simulink model "ackerman_ROS_neural_controller_v2"  (R2023a)
settings: Solver=FixedStepDiscrete  StartTime=0.0  StopTime=200  FixedStep=0.1  RelTol=1e-3
undefined symbols (not defined in the file or in its folder): Angular, Linear
libraries: neural x413, robotlib x15, robotcorelib x1
(part 11 of 17)

== system ackerman_ROS_neural_controller_v2/casi 3 - 15 20 15/Layer 1/IW{1,1} ==
  "pd{1,1}" : Inport  PortDimensions=8  SampleTime=0.1
      mask Display: e = 0.06;c1 = [120 230 180]/255;c2 = ([120 230 180]+0)/(256+128);c3 = ([120 230 180]+128)/(256+128);patch([0 1 1 0],[0 0 1 1],c1);patch([0 1 1 1-e 1-e 0+e],[0 0 1 1-e 0+e 0+e],c2);patch([0 0 1 1-e 0+e 0+e],[0 1 1 1-e 1-e 0+e],c3);plot([0 1 1 0 0],[0 0 1 1 0]);
  "IW{1,1}(1,:)'" : Constant  Value=[2.897737054776072351813809291343204677104949951171875;-0.97777917153495874647006758095812983810901641845703125;-1.95913475138207981984805883257649838924407958984375;3.442897344122934466525975949480198323726654052734375;-7.99002240223826820653130198479630053043365478515625;1.271756533327842220160164288245141506195068359375;5.08245618160992140843745801248587667942047119140625;-9.02719443592735615311539731919765472412109375]
      mask Display: e = 0.06;c1 = [120 150 230]/255;c2 = ([120 150 230]+0)/383;c3 = ([120 150 230]+128)/383;patch([0 1 1 0],[0 0 1 1],c1);patch([0 1 1 1-e 1-e 0+e],[0 0 1 1-e 0+e 0+e],c2);patch([0 0 1 1-e 0+e 0+e],[0 1 1 1-e 1-e 0+e],c3);plot([0 1 1 0 0],[0 0 1 1 0]);disp('Weights');
  "IW{1,1}(10,:)'" : Constant  Value=[-0.82593178229890984454186764196492731571197509765625;2.35210993951447111527386368834413588047027587890625;0.292170459956925199218602529072086326777935028076171875;-1.0114862071536403487215238783392123878002166748046875;-4.12104019955256095641971114673651754856109619140625;-0.81766281683690511528084243764169514179229736328125;1.8519098472877104644140899836202152073383331298828125;-1.116663125058864114436119052697904407978057861328125]
      mask Display: e = 0.06;c1 = [120 150 230]/255;c2 = ([120 150 230]+0)/383;c3 = ([120 150 230]+128)/383;patch([0 1 1 0],[0 0 1 1],c1);patch([0 1 1 1-e 1-e 0+e],[0 0 1 1-e 0+e 0+e],c2);patch([0 0 1 1-e 0+e 0+e],[0 1 1 1-e 1-e 0+e],c3);plot([0 1 1 0 0],[0 0 1 1 0]);disp('Weights');
  "IW{1,1}(11,:)'" : Constant  Value=[-0.078503432809702233807769289342104457318782806396484375;-1.31700463726781347162386737181805074214935302734375;-1.91049666805551243697891550255008041858673095703125;1.4172024682093269376537136849947273731231689453125;-3.09796436612653902642477987683378159999847412109375;-0.98792077372010644875643947671051137149333953857421875;-0.01101359556692830914126357555460344883613288402557373046875;-1.895967746941914722214050925686024129390716552734375]
      mask Display: e = 0.06;c1 = [120 150 230]/255;c2 = ([120 150 230]+0)/383;c3 = ([120 150 230]+128)/383;patch([0 1 1 0],[0 0 1 1],c1);patch([0 1 1 1-e 1-e 0+e],[0 0 1 1-e 0+e 0+e],c2);patch([0 0 1 1-e 0+e 0+e],[0 1 1 1-e 1-e 0+e],c3);plot([0 1 1 0 0],[0 0 1 1 0]);disp('Weights');
  "IW{1,1}(12,:)'" : Constant  Value=[-0.8106197384996172150550819424097426235675811767578125;-0.6227986203077999771693384900572709739208221435546875;1.0411180629325134106011319090612232685089111328125;0.6012357382346260603611654005362652242183685302734375;-1.1876488848888768767864121400634758174419403076171875;-2.475733573131647435872082496643997728824615478515625;-1.7927537050774613458514750163885764777660369873046875;-0.999271370716360962660473887808620929718017578125]
      mask Display: e = 0.06;c1 = [120 150 230]/255;c2 = ([120 150 230]+0)/383;c3 = ([120 150 230]+128)/383;patch([0 1 1 0],[0 0 1 1],c1);patch([0 1 1 1-e 1-e 0+e],[0 0 1 1-e 0+e 0+e],c2);patch([0 0 1 1-e 0+e 0+e],[0 1 1 1-e 1-e 0+e],c3);plot([0 1 1 0 0],[0 0 1 1 0]);disp('Weights');
  "IW{1,1}(13,:)'" : Constant  Value=[1.9200847723387510779247122627566568553447723388671875;1.7864125475128134201696639138390310108661651611328125;-2.619916383345554766748364272643812000751495361328125;-0.368745431713104476756370786461047828197479248046875;-1.7276054344216331681849396773031912744045257568359375;1.2160295695674230298521933946176432073116302490234375;0.266643899945036511045515226214774884283542633056640625;-2.80681458166946651289208602975122630596160888671875]
      mask Display: e = 0.06;c1 = [120 150 230]/255;c2 = ([120 150 230]+0)/383;c3 = ([120 150 230]+128)/383;patch([0 1 1 0],[0 0 1 1],c1);patch([0 1 1 1-e 1-e 0+e],[0 0 1 1-e 0+e 0+e],c2);patch([0 0 1 1-e 0+e 0+e],[0 1 1 1-e 1-e 0+e],c3);plot([0 1 1 0 0],[0 0 1 1 0]);disp('Weights');
  "IW{1,1}(14,:)'" : Constant  Value=[0.9980731449312667535878063063137233257293701171875;-3.114409533087536541273721013567410409450531005859375;0.45617718431620690733296896723913960158824920654296875;-4.31118482402145541954041618737392127513885498046875;0.75844871154216975117634547132183797657489776611328125;4.07356626581029690470359128084965050220489501953125;-0.18504498285524795253564889208064414560794830322265625;0.840293231307919885608725962811149656772613525390625]
      mask Display: e = 0.06;c1 = [120 150 230]/255;c2 = ([120 150 230]+0)/383;c3 = ([120 150 230]+128)/383;patch([0 1 1 0],[0 0 1 1],c1);patch([0 1 1 1-e 1-e 0+e],[0 0 1 1-e 0+e 0+e],c2);patch([0 0 1 1-e 0+e 0+e],[0 1 1 1-e 1-e 0+e],c3);plot([0 1 1 0 0],[0 0 1 1 0]);disp('Weights');
  "IW{1,1}(15,:)'" : Constant  Value=[0.264348557935919270533986491500400006771087646484375;1.6376069116661342572882631429820321500301361083984375;0.54287049402263531927559370160452090203762054443359375;-1.536888279368743059905000336584635078907012939453125;-1.511976681548248269137957322527654469013214111328125;-1.110912669638801641980307977064512670040130615234375;0.323317174054256251114480846808874048292636871337890625;0.49728314679400742459591810984420590102672576904296875]
      mask Display: e = 0.06;c1 = [120 150 230]/255;c2 = ([120 150 230]+0)/383;c3 = ([120 150 230]+128)/383;patch([0 1 1 0],[0 0 1 1],c1);patch([0 1 1 1-e 1-e 0+e],[0 0 1 1-e 0+e 0+e],c2);patch([0 0 1 1-e 0+e 0+e],[0 1 1 1-e 1-e 0+e],c3);plot([0 1 1 0 0],[0 0 1 1 0]);disp('Weights');
  "IW{1,1}(2,:)'" : Constant  Value=[-4.26598336004146716504692449234426021575927734375;-0.0716533501066898559361817433455144055187702178955078125;1.3698494058938184281259964336641132831573486328125;1.0032592579538570642938566379598341882228851318359375;0.1350385776637200996308507683352218009531497955322265625;3.6066214754247578611057178932242095470428466796875;-2.493648707013484955297144551877863705158233642578125;-1.2915573005255687188963520384277217090129852294921875]
      mask Display: e = 0.06;c1 = [120 150 230]/255;c2 = ([120 150 230]+0)/383;c3 = ([120 150 230]+128)/383;patch([0 1 1 0],[0 0 1 1],c1);patch([0 1 1 1-e 1-e 0+e],[0 0 1 1-e 0+e 0+e],c2);patch([0 0 1 1-e 0+e 0+e],[0 1 1 1-e 1-e 0+e],c3);plot([0 1 1 0 0],[0 0 1 1 0]);disp('Weights');
  "IW{1,1}(3,:)'" : Constant  Value=[-2.444535165218435945888586502405814826488494873046875;-1.50490350149213014674387522973120212554931640625;0.06968386498528870987012595605847309343516826629638671875;-0.763333843294209390961668759700842201709747314453125;-3.419767268873754151314869886846281588077545166015625;3.115085244912598749777998818899504840373992919921875;0.60136703915281997101516253678710199892520904541015625;1.74995131625876876313441243837587535381317138671875]
      mask Display: e = 0.06;c1 = [120 150 230]/255;c2 = ([120 150 230]+0)/383;c3 = ([120 150 230]+128)/383;patch([0 1 1 0],[0 0 1 1],c1);patch([0 1 1 1-e 1-e 0+e],[0 0 1 1-e 0+e 0+e],c2);patch([0 0 1 1-e 0+e 0+e],[0 1 1 1-e 1-e 0+e],c3);plot([0 1 1 0 0],[0 0 1 1 0]);disp('Weights');
  "IW{1,1}(4,:)'" : Constant  Value=[-0.64761712625556200340071200116653926670551300048828125;-0.31853889917769662165625277339131571352481842041015625;1.51716786863737151946907033561728894710540771484375;-4.5277687962268426957734845927916467189788818359375;-2.555852630048429663389697452657856047153472900390625;2.557007613553910818637859847513027489185333251953125;0.8989737939253752418977683191769756376743316650390625;0.85350327193705055606187670491635799407958984375]
      mask Display: e = 0.06;c1 = [120 150 230]/255;c2 = ([120 150 230]+0)/383;c3 = ([120 150 230]+128)/383;patch([0 1 1 0],[0 0 1 1],c1);patch([0 1 1 1-e 1-e 0+e],[0 0 1 1-e 0+e 0+e],c2);patch([0 0 1 1-e 0+e 0+e],[0 1 1 1-e 1-e 0+e],c3);plot([0 1 1 0 0],[0 0 1 1 0]);disp('Weights');
  "IW{1,1}(5,:)'" : Constant  Value=[0.0600879788316249496826770837287767790257930755615234375;2.548876161006494722727211410528980195522308349609375;-0.89919509804499553329293348724604584276676177978515625;0.39216783743824390473520224986714310944080352783203125;1.803154797478246695874304350581951439380645751953125;0.670064472196073790399850622634403407573699951171875;0.279308252151045988131983222046983428299427032470703125;-1.9897152695475430750349232766893692314624786376953125]
      mask Display: e = 0.06;c1 = [120 150 230]/255;c2 = ([120 150 230]+0)/383;c3 = ([120 150 230]+128)/383;patch([0 1 1 0],[0 0 1 1],c1);patch([0 1 1 1-e 1-e 0+e],[0 0 1 1-e 0+e 0+e],c2);patch([0 0 1 1-e 0+e 0+e],[0 1 1 1-e 1-e 0+e],c3);plot([0 1 1 0 0],[0 0 1 1 0]);disp('Weights');
  "IW{1,1}(6,:)'" : Constant  Value=[1.516320780958766878399046618142165243625640869140625;-1.15730560900975998350759255117736756801605224609375;0.458524114660376624907911491391132585704326629638671875;-1.102990345663160010047931791632436215877532958984375;2.2751191767257754605680020176805555820465087890625;0.26970804091846589667369471499114297330379486083984375;0.009118671069833252096348275017589912749826908111572265625;0.030751765387002298612895145879519986920058727264404296875]
      mask Display: e = 0.06;c1 = [120 150 230]/255;c2 = ([120 150 230]+0)/383;c3 = ([120 150 230]+128)/383;patch([0 1 1 0],[0 0 1 1],c1);patch([0 1 1 1-e 1-e 0+e],[0 0 1 1-e 0+e 0+e],c2);patch([0 0 1 1-e 0+e 0+e],[0 1 1 1-e 1-e 0+e],c3);plot([0 1 1 0 0],[0 0 1 1 0]);disp('Weights');
  "IW{1,1}(7,:)'" : Constant  Value=[1.0256630959773380684652011041180230677127838134765625;0.953736010400195066694095658021979033946990966796875;0.91140415232379068388723908356041647493839263916015625;0.07112913381762824005516421266293036751449108123779296875;1.7300742608625514495912511847564019262790679931640625;-1.3492253267064329147473245029686950147151947021484375;1.091559740272355583101671072654426097869873046875;0.1343110570666319336652350102667696774005889892578125]
      mask Display: e = 0.06;c1 = [120 150 230]/255;c2 = ([120 150 230]+0)/383;c3 = ([120 150 230]+128)/383;patch([0 1 1 0],[0 0 1 1],c1);patch([0 1 1 1-e 1-e 0+e],[0 0 1 1-e 0+e 0+e],c2);patch([0 0 1 1-e 0+e 0+e],[0 1 1 1-e 1-e 0+e],c3);plot([0 1 1 0 0],[0 0 1 1 0]);disp('Weights');
  "IW{1,1}(8,:)'" : Constant  Value=[-0.46823002994979656676832746597938239574432373046875;-2.389488306025070674110111212939955294132232666015625;1.19212611072083252139464093488641083240509033203125;0.203108224876829390748156356494291685521602630615234375;-3.12759889820417225081428114208392798900604248046875;-4.1826406226244738917330323602072894573211669921875;-0.83564532349110642872602738862042315304279327392578125;0.24560268558538178584882416544132865965366363525390625]
      mask Display: e = 0.06;c1 = [120 150 230]/255;c2 = ([120 150 230]+0)/383;c3 = ([120 150 230]+128)/383;patch([0 1 1 0],[0 0 1 1],c1);patch([0 1 1 1-e 1-e 0+e],[0 0 1 1-e 0+e 0+e],c2);patch([0 0 1 1-e 0+e 0+e],[0 1 1 1-e 1-e 0+e],c3);plot([0 1 1 0 0],[0 0 1 1 0]);disp('Weights');
  "IW{1,1}(9,:)'" : Constant  Value=[0.1263911266086849838341521490292507223784923553466796875;0.0566874449298560012522329998319037258625030517578125;1.8401514119086339604791646706871688365936279296875;0.528937864859507111958691893960349261760711669921875;3.9851213758785686280816662474535405635833740234375;-1.5845796502176010545070994339766912162303924560546875;0.82335138653403949771103498278534971177577972412109375;-0.1356210234756699828384540751358144916594028472900390625]
      mask Display: e = 0.06;c1 = [120 150 230]/255;c2 = ([120 150 230]+0)/383;c3 = ([120 150 230]+128)/383;patch([0 1 1 0],[0 0 1 1],c1);patch([0 1 1 1-e 1-e 0+e],[0 0 1 1-e 0+e 0+e],c2);patch([0 0 1 1-e 0+e 0+e],[0 1 1 1-e 1-e 0+e],c3);plot([0 1 1 0 0],[0 0 1 1 0]);disp('Weights');
  Mux : Mux  Inputs=15
      mask Display: e = 0.06;c1 = [120 150 230]/255;c2 = ([120 150 230]+0)/383;c3 = ([120 150 230]+128)/383;patch([0 1 1 0],[0 0 1 1],c1);patch([0 1 1 1-e 1-e 0+e],[0 0 1 1-e 0+e 0+e],c2);patch([0 0 1 1-e 0+e 0+e],[0 1 1 1-e 1-e 0+e],c3);plot([0 1 1 0 0],[0 0 1 1 0]);disp('Mux');
  dotprod{1..15} (15 alike) : neural/Weight Functions/dotprod
  "iz{1,1}" : Outport
      mask Display: e = 0.06;c1 = [120 230 180]/255;c2 = ([120 230 180]+0)/(256+128);c3 = ([120 230 180]+128)/(256+128);patch([0 1 1 0],[0 0 1 1],c1);patch([0 1 1 1-e 1-e 0+e],[0 0 1 1-e 0+e 0+e],c2);patch([0 0 1 1-e 0+e 0+e],[0 1 1 1-e 1-e 0+e],c3);plot([0 1 1 0 0],[0 0 1 1 0]);
  wires:
  "IW{1,1}(1,:)'"/1 -> dotprod1/1
  "pd{1,1}"/1 -> dotprod1/2, dotprod2/2, dotprod3/2, dotprod4/2, dotprod5/2, dotprod6/2, dotprod7/2, dotprod8/2, dotprod9/2, dotprod10/2, dotprod11/2, dotprod12/2, dotprod13/2, dotprod14/2, dotprod15/2
  dotprod1/1 -> Mux/1
  "IW{1,1}(2,:)'"/1 -> dotprod2/1
  dotprod2/1 -> Mux/2
  "IW{1,1}(3,:)'"/1 -> dotprod3/1
  dotprod3/1 -> Mux/3
  "IW{1,1}(4,:)'"/1 -> dotprod4/1
  dotprod4/1 -> Mux/4
  "IW{1,1}(5,:)'"/1 -> dotprod5/1
  dotprod5/1 -> Mux/5
  "IW{1,1}(6,:)'"/1 -> dotprod6/1
  dotprod6/1 -> Mux/6
  "IW{1,1}(7,:)'"/1 -> dotprod7/1
  dotprod7/1 -> Mux/7
  "IW{1,1}(8,:)'"/1 -> dotprod8/1
  dotprod8/1 -> Mux/8
  "IW{1,1}(9,:)'"/1 -> dotprod9/1
  dotprod9/1 -> Mux/9
  "IW{1,1}(10,:)'"/1 -> dotprod10/1
  dotprod10/1 -> Mux/10
  "IW{1,1}(11,:)'"/1 -> dotprod11/1
  dotprod11/1 -> Mux/11
  "IW{1,1}(12,:)'"/1 -> dotprod12/1
  dotprod12/1 -> Mux/12
  "IW{1,1}(13,:)'"/1 -> dotprod13/1
  dotprod13/1 -> Mux/13
  "IW{1,1}(14,:)'"/1 -> dotprod14/1
  dotprod14/1 -> Mux/14
  "IW{1,1}(15,:)'"/1 -> dotprod15/1
  dotprod15/1 -> Mux/15
  Mux/1 -> "iz{1,1}"/1

== system ackerman_ROS_neural_controller_v2/casi 3 - 15 20 15/Layer 2/Delays 1 ==
  "p{2}" : Inport  PortDimensions=15  SampleTime=0.1
      mask Display: e = 0.06;c1 = [120 230 180]/255;c2 = ([120 230 180]+0)/(256+128);c3 = ([120 230 180]+128)/(256+128);patch([0 1 1 0],[0 0 1 1],c1);patch([0 1 1 1-e 1-e 0+e],[0 0 1 1-e 0+e 0+e],c2);patch([0 0 1 1-e 0+e 0+e],[0 1 1 1-e 1-e 0+e],c3);plot([0 1 1 0 0],[0 0 1 1 0]);
  mux : Mux  Inputs=1
      mask Display: e = 0.06;c1 = [120 150 230]/255;c2 = ([120 150 230]+0)/383;c3 = ([120 150 230]+128)/383;patch([0 1 1 0],[0 0 1 1],c1);patch([0 1 1 1-e 1-e 0+e],[0 0 1 1-e 0+e 0+e],c2);patch([0 0 1 1-e 0+e 0+e],[0 1 1 1-e 1-e 0+e],c3);plot([0 1 1 0 0],[0 0 1 1 0]);disp('Mux')
  "pd{2,1}" : Outport
      mask Display: e = 0.06;c1 = [120 230 180]/255;c2 = ([120 230 180]+0)/(256+128);c3 = ([120 230 180]+128)/(256+128);patch([0 1 1 0],[0 0 1 1],c1);patch([0 1 1 1-e 1-e 0+e],[0 0 1 1-e 0+e 0+e],c2);patch([0 0 1 1-e 0+e 0+e],[0 1 1 1-e 1-e 0+e],c3);plot([0 1 1 0 0],[0 0 1 1 0]);
  wires:
  "p{2}"/1 -> mux/1
  mux/1 -> "pd{2,1}"/1

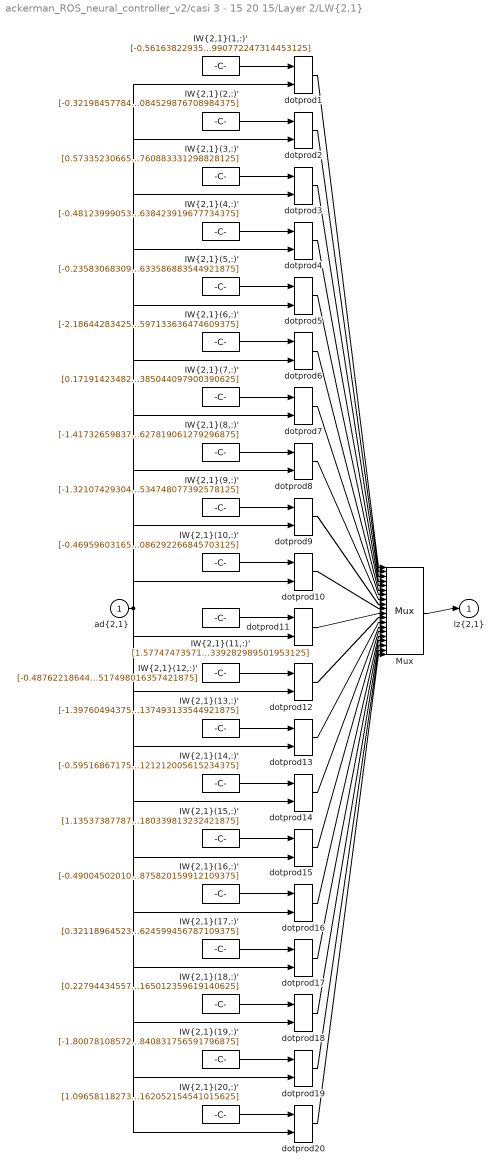
== system ackerman_ROS_neural_controller_v2/casi 3 - 15 20 15/Layer 2/LW{2,1} ==
  "ad{2,1}" : Inport  PortDimensions=15  SampleTime=0.1
      mask Display: e = 0.06;c1 = [120 230 180]/255;c2 = ([120 230 180]+0)/(256+128);c3 = ([120 230 180]+128)/(256+128);patch([0 1 1 0],[0 0 1 1],c1);patch([0 1 1 1-e 1-e 0+e],[0 0 1 1-e 0+e 0+e],c2);patch([0 0 1 1-e 0+e 0+e],[0 1 1 1-e 1-e 0+e],c3);plot([0 1 1 0 0],[0 0 1 1 0]);
  "IW{2,1}(1,:)'" : Constant  Value=[-0.56163822935183393969538201417890377342700958251953125;0.245452610051165975857401235771249048411846160888671875;-0.377698889868788800772136937666800804436206817626953125;-0.68762869818237515318060104618780314922332763671875;0.40400799476497561979471129234298132359981536865234375;0.68723151557078576701087513356469571590423583984375;0.50809930187312291050005796932964585721492767333984375;-1.6550057236130319981981529053882695734500885009765625;0.400536181872844954110490789389587007462978363037109375;0.9964717790251331752671148933586664497852325439453125;0.0679652649393227281660045946409809403121471405029296875;-0.99403156544476967138024292580666951835155487060546875;0.01500446131223251954034392241510431631468236446380615234375;-0.06991876875524201395695200744739850051701068878173828125;0.780413619069737496403149634716100990772247314453125]
      mask Display: e = 0.06;c1 = [120 150 230]/255;c2 = ([120 150 230]+0)/383;c3 = ([120 150 230]+128)/383;patch([0 1 1 0],[0 0 1 1],c1);patch([0 1 1 1-e 1-e 0+e],[0 0 1 1-e 0+e 0+e],c2);patch([0 0 1 1-e 0+e 0+e],[0 1 1 1-e 1-e 0+e],c3);plot([0 1 1 0 0],[0 0 1 1 0]);disp('weights');
  "IW{2,1}(10,:)'" : Constant  Value=[-0.469596031658941204245394374083844013512134552001953125;1.964028913619128235978905649972148239612579345703125;0.63289993982047543230606834185891784727573394775390625;-0.412008432682525349566304839754593558609485626220703125;-0.53118016805264023361132785794325172901153564453125;3.443822119182487373478807057836093008518218994140625;-0.2461500747600740834908350507248542271554470062255859375;1.17739031454758613648436949006281793117523193359375;0.26849885847382648496051160691422410309314727783203125;2.551982968568425658162368563353084027767181396484375;0.1488598365930947908797321588281192816793918609619140625;0.981327233075227400860285342787392437458038330078125;-0.472821390015247089433358951282571069896221160888671875;-0.0187855024166666585705431913311258540488779544830322265625;1.6333664356874006973185942115378566086292266845703125]
      mask Display: e = 0.06;c1 = [120 150 230]/255;c2 = ([120 150 230]+0)/383;c3 = ([120 150 230]+128)/383;patch([0 1 1 0],[0 0 1 1],c1);patch([0 1 1 1-e 1-e 0+e],[0 0 1 1-e 0+e 0+e],c2);patch([0 0 1 1-e 0+e 0+e],[0 1 1 1-e 1-e 0+e],c3);plot([0 1 1 0 0],[0 0 1 1 0]);disp('weights');
  "IW{2,1}(11,:)'" : Constant  Value=[1.5774747357148506399227017027442343533039093017578125;1.31591759457128798516123424633406102657318115234375;1.3082425648586981647980564957833848893642425537109375;1.8159158316652928011336598501657135784626007080078125;-1.0542224907578108261674287859932519495487213134765625;1.538409972199835440420656595961190760135650634765625;-0.93064977698365092262378084342344664037227630615234375;-0.804425007696444094307253180886618793010711669921875;0.32814276677999121289985851035453379154205322265625;1.5353571917339225993970330819138325750827789306640625;0.87847183842192622105216059935628436505794525146484375;-0.061412736428054982840141207134365686215460300445556640625;0.08139325792860295505359857770599774084985256195068359375;0.358563222723859598151108230013051070272922515869140625;0.60452773396042946973949483435717411339282989501953125]
      mask Display: e = 0.06;c1 = [120 150 230]/255;c2 = ([120 150 230]+0)/383;c3 = ([120 150 230]+128)/383;patch([0 1 1 0],[0 0 1 1],c1);patch([0 1 1 1-e 1-e 0+e],[0 0 1 1-e 0+e 0+e],c2);patch([0 0 1 1-e 0+e 0+e],[0 1 1 1-e 1-e 0+e],c3);plot([0 1 1 0 0],[0 0 1 1 0]);disp('weights');
  "IW{2,1}(12,:)'" : Constant  Value=[-0.48762218644485055829562725193682126700878143310546875;0.328876498199026479074547069103573448956012725830078125;-0.597352360147869188011782171088270843029022216796875;0.53534216932835698710135829969658516347408294677734375;1.6950029674032667248440020557609386742115020751953125;0.9126979466616518266164348460733890533447265625;-0.4831878795116864022674008083413355052471160888671875;2.8415640766889307400333564146421849727630615234375;-1.230805250099656245055257386411540210247039794921875;1.29942734563329143071541693643666803836822509765625;0.67789586952500757721651325482525862753391265869140625;-0.7393149068396607237474427165579982101917266845703125;-0.8306390478651810571619762413320131599903106689453125;1.7719520385174167831365821257350035011768341064453125;-1.6650125512326290344589097003336064517498016357421875]
      mask Display: e = 0.06;c1 = [120 150 230]/255;c2 = ([120 150 230]+0)/383;c3 = ([120 150 230]+128)/383;patch([0 1 1 0],[0 0 1 1],c1);patch([0 1 1 1-e 1-e 0+e],[0 0 1 1-e 0+e 0+e],c2);patch([0 0 1 1-e 0+e 0+e],[0 1 1 1-e 1-e 0+e],c3);plot([0 1 1 0 0],[0 0 1 1 0]);disp('weights');
  "IW{2,1}(13,:)'" : Constant  Value=[-1.397604943750206274444281007163226604461669921875;-1.0930238364841919906922385052894242107868194580078125;-0.434360790054279244376544966144138015806674957275390625;-0.5909797323172616412279012365615926682949066162109375;0.90278744353159179336643092028680257499217987060546875;-0.48525826816891537429654590596328489482402801513671875;-0.1928533926542131127224166675659944303333759307861328125;1.0427414421290752688520342417177744209766387939453125;2.09104540100165170457557906047441065311431884765625;1.2284581799702951609987167103099636733531951904296875;1.1097882783759527303146796839428134262561798095703125;0.511566753687448194654052713303826749324798583984375;-2.02906487925908773917171856737695634365081787109375;-1.1747520683242107519816954663838259875774383544921875;0.66003641258386103185529236725415103137493133544921875]
      mask Display: e = 0.06;c1 = [120 150 230]/255;c2 = ([120 150 230]+0)/383;c3 = ([120 150 230]+128)/383;patch([0 1 1 0],[0 0 1 1],c1);patch([0 1 1 1-e 1-e 0+e],[0 0 1 1-e 0+e 0+e],c2);patch([0 0 1 1-e 0+e 0+e],[0 1 1 1-e 1-e 0+e],c3);plot([0 1 1 0 0],[0 0 1 1 0]);disp('weights');
  "IW{2,1}(14,:)'" : Constant  Value=[-0.595168671758967260387862552306614816188812255859375;1.509010237064945414431349490769207477569580078125;-0.96671320639537483554448726863483898341655731201171875;2.706437334121316151680503026000224053859710693359375;0.85733564653706795244403338074334897100925445556640625;-0.87513032385332767404406695277430117130279541015625;2.521230549385313768340211026952601969242095947265625;1.536037438834628954253957999753765761852264404296875;2.01164529118437673815833477419801056385040283203125;-1.1471441599588485527050352175137959420680999755859375;-0.0737940849847644464443163769828970544040203094482421875;0.88401859050396358608026048386818729341030120849609375;-0.98105258755058410979899008452775888144969940185546875;-0.458262491412897265963266590915736742317676544189453125;-5.92325886066728823919902424677275121212005615234375]
      mask Display: e = 0.06;c1 = [120 150 230]/255;c2 = ([120 150 230]+0)/383;c3 = ([120 150 230]+128)/383;patch([0 1 1 0],[0 0 1 1],c1);patch([0 1 1 1-e 1-e 0+e],[0 0 1 1-e 0+e 0+e],c2);patch([0 0 1 1-e 0+e 0+e],[0 1 1 1-e 1-e 0+e],c3);plot([0 1 1 0 0],[0 0 1 1 0]);disp('weights');
  "IW{2,1}(15,:)'" : Constant  Value=[1.1353738778705046996719829621724784374237060546875;2.544503291133388689360117496107704937458038330078125;-0.2017096647714138324403165825060568749904632568359375;1.169534184688194589085696861729957163333892822265625;-0.473076056622592222566936470684595406055450439453125;-0.1403074579502983088019618662656284868717193603515625;-0.016696044346578738093445082313337479718029499053955078125;-0.9715453026856122331622600540868006646633148193359375;0.7348332962173065308064678902155719697475433349609375;2.717485620282661162860904369154013693332672119140625;-1.8514811187874453679569342057220637798309326171875;0.0785364932365222312427022188785485923290252685546875;-1.0395875618079244429026175566832534968852996826171875;-0.79087471733962522169036901686922647058963775634765625;-1.99363520319415510329008611734025180339813232421875]
      mask Display: e = 0.06;c1 = [120 150 230]/255;c2 = ([120 150 230]+0)/383;c3 = ([120 150 230]+128)/383;patch([0 1 1 0],[0 0 1 1],c1);patch([0 1 1 1-e 1-e 0+e],[0 0 1 1-e 0+e 0+e],c2);patch([0 0 1 1-e 0+e 0+e],[0 1 1 1-e 1-e 0+e],c3);plot([0 1 1 0 0],[0 0 1 1 0]);disp('weights');
  "IW{2,1}(16,:)'" : Constant  Value=[-0.490045020107930551223063275756430812180042266845703125;0.35048308998360067079147484037093818187713623046875;-0.29677847859899575411191108287312090396881103515625;0.303808900779805546310541330967680551111698150634765625;-0.006732479297560066411332257985122851096093654632568359375;-0.1901635060205711102998549222320434637367725372314453125;-0.69393242785902276015264078523614443838596343994140625;-0.342819841103145339644697742187418043613433837890625;0.447241150252011998578183238350902684032917022705078125;-0.4730642440810524096406197713804431259632110595703125;0.429529221821453532914603101744432933628559112548828125;0.67936327673356888823263943777419626712799072265625;0.97513320129287162085773843500646762549877166748046875;-0.1714178569641091887110206926081445999443531036376953125;-1.537248919602196561839946298277936875820159912109375]
      mask Display: e = 0.06;c1 = [120 150 230]/255;c2 = ([120 150 230]+0)/383;c3 = ([120 150 230]+128)/383;patch([0 1 1 0],[0 0 1 1],c1);patch([0 1 1 1-e 1-e 0+e],[0 0 1 1-e 0+e 0+e],c2);patch([0 0 1 1-e 0+e 0+e],[0 1 1 1-e 1-e 0+e],c3);plot([0 1 1 0 0],[0 0 1 1 0]);disp('weights');
  "IW{2,1}(17,:)'" : Constant  Value=[0.3211896452377012156631508332793600857257843017578125;-0.951152018348393024638198767206631600856781005859375;-1.0162950319598060833214958620374090969562530517578125;0.213405770054723331607959835309884510934352874755859375;-0.12557524981967116417536090011708438396453857421875;-0.92525668302915498042438002812559716403484344482421875;0.264687545270491597637629865857888944447040557861328125;0.341360691469928756447416162700392305850982666015625;0.398342129560288193967920733484788797795772552490234375;-0.43925310856936106151948706610710360109806060791015625;-0.32212143647492752496219736713101156055927276611328125;-1.2536628119730306440970935000223107635974884033203125;-0.76882931437409152142237189764273352921009063720703125;0.87751958026946941249235578652587719261646270751953125;0.96558691091337711664976950487471185624599456787109375]
      mask Display: e = 0.06;c1 = [120 150 230]/255;c2 = ([120 150 230]+0)/383;c3 = ([120 150 230]+128)/383;patch([0 1 1 0],[0 0 1 1],c1);patch([0 1 1 1-e 1-e 0+e],[0 0 1 1-e 0+e 0+e],c2);patch([0 0 1 1-e 0+e 0+e],[0 1 1 1-e 1-e 0+e],c3);plot([0 1 1 0 0],[0 0 1 1 0]);disp('weights');
  "IW{2,1}(18,:)'" : Constant  Value=[0.2279443455771786031238690384270739741623401641845703125;0.2190624194632964372164707356205326505005359649658203125;-0.484047560658517783682697199765243567526340484619140625;-1.4459444695820753423731730435974895954132080078125;0.64338800149315467091781783892656676471233367919921875;-1.0457896595276470197433127395925112068653106689453125;0.53870688324349202957819215953350067138671875;-0.88840962740939655173377786923083476722240447998046875;-0.032228735377791827010351966009693569503724575042724609375;1.2682066824984212782823078669025562703609466552734375;-0.05978913659068153807485401785015710629522800445556640625;1.3288624932237558251557629773742519319057464599609375;-0.350162441069049423791881281431415118277072906494140625;-1.008688661839455047442015711567364633083343505859375;0.185662207021203118362251416328945197165012359619140625]
      mask Display: e = 0.06;c1 = [120 150 230]/255;c2 = ([120 150 230]+0)/383;c3 = ([120 150 230]+128)/383;patch([0 1 1 0],[0 0 1 1],c1);patch([0 1 1 1-e 1-e 0+e],[0 0 1 1-e 0+e 0+e],c2);patch([0 0 1 1-e 0+e 0+e],[0 1 1 1-e 1-e 0+e],c3);plot([0 1 1 0 0],[0 0 1 1 0]);disp('weights');
  "IW{2,1}(19,:)'" : Constant  Value=[-1.8007810857265227344470304160495288670063018798828125;1.1274205090982416521683262544684112071990966796875;1.8818893125960347578740083918091841042041778564453125;-0.73769150106170677805295099460636265575885772705078125;-4.56188115457599874247307525365613400936126708984375;0.96172126887003062112313500620075501501560211181640625;-0.418434002804122684437970747239887714385986328125;-1.009698878513926700861702556721866130828857421875;1.5760574723669920071955630191951058804988861083984375;-0.1302369200222082967766112915342091582715511322021484375;-0.367498366488594907508513642824254930019378662109375;1.75476493300579949874418161925859749317169189453125;0.489786600447615960707281601571594364941120147705078125;-0.8969680273044906559931632727966643869876861572265625;-1.0615610455301396353178233766811899840831756591796875]
      mask Display: e = 0.06;c1 = [120 150 230]/255;c2 = ([120 150 230]+0)/383;c3 = ([120 150 230]+128)/383;patch([0 1 1 0],[0 0 1 1],c1);patch([0 1 1 1-e 1-e 0+e],[0 0 1 1-e 0+e 0+e],c2);patch([0 0 1 1-e 0+e 0+e],[0 1 1 1-e 1-e 0+e],c3);plot([0 1 1 0 0],[0 0 1 1 0]);disp('weights');
  "IW{2,1}(2,:)'" : Constant  Value=[-0.32198457784391099067988761817105114459991455078125;0.1973043757795246710973202652894542552530765533447265625;1.2233656872245040059254961306578479707241058349609375;-0.03882472774771596191190070612719864584505558013916015625;-0.301611555539175235640669825443183071911334991455078125;0.395294411528984312997891947816242463886737823486328125;-0.061911653933364674262662674664170481264591217041015625;0.54557012874814125868994096890673972666263580322265625;0.1248663627079501237115977119174203835427761077880859375;0.8390437777058890045367434140644036233425140380859375;-0.8827347091295065784066764535964466631412506103515625;-0.482814374847474636620603405390284024178981781005859375;-0.004982110850706436382118180716815913910977542400360107421875;0.297683903332398802632496881415136158466339111328125;-1.06905706048156812215665922849439084529876708984375]
      mask Display: e = 0.06;c1 = [120 150 230]/255;c2 = ([120 150 230]+0)/383;c3 = ([120 150 230]+128)/383;patch([0 1 1 0],[0 0 1 1],c1);patch([0 1 1 1-e 1-e 0+e],[0 0 1 1-e 0+e 0+e],c2);patch([0 0 1 1-e 0+e 0+e],[0 1 1 1-e 1-e 0+e],c3);plot([0 1 1 0 0],[0 0 1 1 0]);disp('weights');
  "IW{2,1}(20,:)'" : Constant  Value=[1.096581182732693005021928911446593701839447021484375;-1.62109365647088754514015818131156265735626220703125;-0.79258998242899270092465258130687288939952850341796875;-0.351961894963530974589360766913159750401973724365234375;1.6386434258634146043931423264439217746257781982421875;-2.08164245601561770371290549519471824169158935546875;-0.6236274815186992892535045029944740235805511474609375;-0.421730319480988213864947056208620779216289520263671875;-0.8698551994897794070737973015638999640941619873046875;-0.540930402141860167120057667489163577556610107421875;0.91160404562427055363826866596355102956295013427734375;0.14694630518057516521679417564882896840572357177734375;1.4374032545034001184802718853461556136608123779296875;-0.048312194119506081391168805794222862459719181060791015625;-0.66623985436569965745690069525153376162052154541015625]
      mask Display: e = 0.06;c1 = [120 150 230]/255;c2 = ([120 150 230]+0)/383;c3 = ([120 150 230]+128)/383;patch([0 1 1 0],[0 0 1 1],c1);patch([0 1 1 1-e 1-e 0+e],[0 0 1 1-e 0+e 0+e],c2);patch([0 0 1 1-e 0+e 0+e],[0 1 1 1-e 1-e 0+e],c3);plot([0 1 1 0 0],[0 0 1 1 0]);disp('weights');
  "IW{2,1}(3,:)'" : Constant  Value=[0.5733523066513186439152605089475400745868682861328125;-2.79022839717246284862994798459112644195556640625;-1.50488242776033853687067676219157874584197998046875;0.314987098052309288931382980081252753734588623046875;0.96615414990402281869563694272073917090892791748046875;0.049715463903150160229760246011210256256163120269775390625;-3.45320499749016018853353671147488057613372802734375;-1.0678897186616638226297482106019742786884307861328125;1.477959833227803443378434167243540287017822265625;1.183433401868228873610178197850473225116729736328125;-1.20317382600841416007142470334656536579132080078125;-0.30197360945173212787295824455213733017444610595703125;-0.01041284887243107241949768848598978365771472454071044921875;-0.447432787017421118580529082464636303484439849853515625;-0.186417589750945911220014750142581760883331298828125]
      mask Display: e = 0.06;c1 = [120 150 230]/255;c2 = ([120 150 230]+0)/383;c3 = ([120 150 230]+128)/383;patch([0 1 1 0],[0 0 1 1],c1);patch([0 1 1 1-e 1-e 0+e],[0 0 1 1-e 0+e 0+e],c2);patch([0 0 1 1-e 0+e 0+e],[0 1 1 1-e 1-e 0+e],c3);plot([0 1 1 0 0],[0 0 1 1 0]);disp('weights');
  "IW{2,1}(4,:)'" : Constant  Value=[-0.481239990536924011621522367931902408599853515625;-0.6602672991926734624712480581365525722503662109375;0.473998241701680311788180688381544314324855804443359375;-0.69961086122611437776441789537784643471240997314453125;0.69680259372673158946298599403235130012035369873046875;0.1557231667111025341654340081731788814067840576171875;-0.0629796555406990365977293322430341504514217376708984375;0.77446614968832261372000402843696065247058868408203125;0.0100079632011082740594698492486713803373277187347412109375;-0.10308173179035241828760405269349575974047183990478515625;0.3459812314341437211595575718092732131481170654296875;0.75550833601784450621607902576215565204620361328125;0.032545046732226044772229300860999501310288906097412109375;-0.3316508767213182107269631160306744277477264404296875;-0.90146390938654741287194838150753639638423919677734375]
      mask Display: e = 0.06;c1 = [120 150 230]/255;c2 = ([120 150 230]+0)/383;c3 = ([120 150 230]+128)/383;patch([0 1 1 0],[0 0 1 1],c1);patch([0 1 1 1-e 1-e 0+e],[0 0 1 1-e 0+e 0+e],c2);patch([0 0 1 1-e 0+e 0+e],[0 1 1 1-e 1-e 0+e],c3);plot([0 1 1 0 0],[0 0 1 1 0]);disp('weights');
  "IW{2,1}(5,:)'" : Constant  Value=[-0.2358306830958407374065899375636945478618144989013671875;0.5471805702598613319054265957674942910671234130859375;-0.88823215691268575522343553529935888946056365966796875;-0.38321354261398676843697330696159042418003082275390625;-2.33776688046363378958858447731472551822662353515625;4.82814920808915193362054196768440306186676025390625;-0.4697607447236651356803349699475802481174468994140625;1.2007763226738299433549173045321367681026458740234375;-2.389021249038371319528550884569995105266571044921875;0.8893079951731415189186691350187174975872039794921875;-1.13463739616270942178744007833302021026611328125;-0.759979666560974376210424452438019216060638427734375;1.51220598478428858157940339879132807254791259765625;0.75030538027982773829904772355803288519382476806640625;-3.092896581810016254365791610325686633586883544921875]
      mask Display: e = 0.06;c1 = [120 150 230]/255;c2 = ([120 150 230]+0)/383;c3 = ([120 150 230]+128)/383;patch([0 1 1 0],[0 0 1 1],c1);patch([0 1 1 1-e 1-e 0+e],[0 0 1 1-e 0+e 0+e],c2);patch([0 0 1 1-e 0+e 0+e],[0 1 1 1-e 1-e 0+e],c3);plot([0 1 1 0 0],[0 0 1 1 0]);disp('weights');
  "IW{2,1}(6,:)'" : Constant  Value=[-2.186442834252392941607467946596443653106689453125;-0.03642462591925432757733460675808601081371307373046875;2.32499239862787820953826667391695082187652587890625;-0.718342085904414062724754330702126026153564453125;1.6926651505906622485753132423269562423229217529296875;-0.8547658507198854227482343048905022442340850830078125;-0.30935172443853964363569275519694201648235321044921875;-0.2758511329421426960806229544687084853649139404296875;1.0985261994478443536848999428912065923213958740234375;3.16522439823226786614895900129340589046478271484375;0.147256777991448206677205234882421791553497314453125;0.46408565523117328854851848518592305481433868408203125;1.0291732926077836740574866780661977827548980712890625;0.172782794146276452718069549518986605107784271240234375;-1.3526986943967107546171746434993110597133636474609375]
      mask Display: e = 0.06;c1 = [120 150 230]/255;c2 = ([120 150 230]+0)/383;c3 = ([120 150 230]+128)/383;patch([0 1 1 0],[0 0 1 1],c1);patch([0 1 1 1-e 1-e 0+e],[0 0 1 1-e 0+e 0+e],c2);patch([0 0 1 1-e 0+e 0+e],[0 1 1 1-e 1-e 0+e],c3);plot([0 1 1 0 0],[0 0 1 1 0]);disp('weights');
  "IW{2,1}(7,:)'" : Constant  Value=[0.1719142348290966515467204089873121120035648345947265625;0.45120324698051472722681864979676902294158935546875;-0.75231635981951427982750146838952787220478057861328125;1.8129897329620536794436702621169388294219970703125;-1.4778298522470196818545673522748984396457672119140625;-1.953718055616802562468592441291548311710357666015625;0.965566589141327202838738230639137327671051025390625;0.52097490851912764409092915229848586022853851318359375;0.95812585212619560959268483202322386205196380615234375;-1.9821255985650463316005698288790881633758544921875;1.868368621496311110519172871136106550693511962890625;-1.597780718779968633924681853386573493480682373046875;2.030521169982075324611514588468708097934722900390625;-0.032483064289437042770902763777485233731567859649658203125;-2.51619458131580930881909807794727385044097900390625]
      mask Display: e = 0.06;c1 = [120 150 230]/255;c2 = ([120 150 230]+0)/383;c3 = ([120 150 230]+128)/383;patch([0 1 1 0],[0 0 1 1],c1);patch([0 1 1 1-e 1-e 0+e],[0 0 1 1-e 0+e 0+e],c2);patch([0 0 1 1-e 0+e 0+e],[0 1 1 1-e 1-e 0+e],c3);plot([0 1 1 0 0],[0 0 1 1 0]);disp('weights');
  "IW{2,1}(8,:)'" : Constant  Value=[-1.4173265983704952386545983245014213025569915771484375;0.759505216114494174917126656509935855865478515625;0.08700579767931611308018347017423366196453571319580078125;0.90251938594767311396793729727505706250667572021484375;-0.10302356674944633530000004384419298730790615081787109375;-0.72771523277017891029316842832486145198345184326171875;0.9636772470330681183980914283893071115016937255859375;-1.412627442167801117278713718405924737453460693359375;0.0678023763816388014280533980127074755728244781494140625;-0.86501775933870417301108091123751364648342132568359375;0.1614053782787632507211839083538507111370563507080078125;-0.84874665066786436629087120309122838079929351806640625;-2.167752502921040491656867743586190044879913330078125;0.7972136666608502508779565687291324138641357421875;1.0401214708131110153743748014676384627819061279296875]
      mask Display: e = 0.06;c1 = [120 150 230]/255;c2 = ([120 150 230]+0)/383;c3 = ([120 150 230]+128)/383;patch([0 1 1 0],[0 0 1 1],c1);patch([0 1 1 1-e 1-e 0+e],[0 0 1 1-e 0+e 0+e],c2);patch([0 0 1 1-e 0+e 0+e],[0 1 1 1-e 1-e 0+e],c3);plot([0 1 1 0 0],[0 0 1 1 0]);disp('weights');
  "IW{2,1}(9,:)'" : Constant  Value=[-1.32107429304930246161120521719567477703094482421875;-1.9313060512476714070118077870574779808521270751953125;-1.0185027993430380011119495975435711443424224853515625;0.0704284224221078669625484280913951806724071502685546875;-1.042824677774083053094500428414903581142425537109375;0.2932625305508718138725043900194577872753143310546875;0.253166395198550497891432087271823547780513763427734375;0.155737473775058921088287888778722845017910003662109375;1.7103735428391819706206433693296276032924652099609375;-2.30891283988711393249104730784893035888671875;0.591387801979964766729835901060141623020172119140625;-0.2420862926498229816818508197684423066675662994384765625;-1.81393122853091171009509707801043987274169921875;-1.2622931498818197315614497711067087948322296142578125;-1.89661486432261927603803997044451534748077392578125]
      mask Display: e = 0.06;c1 = [120 150 230]/255;c2 = ([120 150 230]+0)/383;c3 = ([120 150 230]+128)/383;patch([0 1 1 0],[0 0 1 1],c1);patch([0 1 1 1-e 1-e 0+e],[0 0 1 1-e 0+e 0+e],c2);patch([0 0 1 1-e 0+e 0+e],[0 1 1 1-e 1-e 0+e],c3);plot([0 1 1 0 0],[0 0 1 1 0]);disp('weights');
  Mux : Mux  Inputs=20
      mask Display: e = 0.06;c1 = [120 150 230]/255;c2 = ([120 150 230]+0)/383;c3 = ([120 150 230]+128)/383;patch([0 1 1 0],[0 0 1 1],c1);patch([0 1 1 1-e 1-e 0+e],[0 0 1 1-e 0+e 0+e],c2);patch([0 0 1 1-e 0+e 0+e],[0 1 1 1-e 1-e 0+e],c3);plot([0 1 1 0 0],[0 0 1 1 0]);disp('Mux');
  dotprod{1..20} (20 alike) : neural/Weight Functions/dotprod
  "lz{2,1}" : Outport
      mask Display: e = 0.06;c1 = [120 230 180]/255;c2 = ([120 230 180]+0)/(256+128);c3 = ([120 230 180]+128)/(256+128);patch([0 1 1 0],[0 0 1 1],c1);patch([0 1 1 1-e 1-e 0+e],[0 0 1 1-e 0+e 0+e],c2);patch([0 0 1 1-e 0+e 0+e],[0 1 1 1-e 1-e 0+e],c3);plot([0 1 1 0 0],[0 0 1 1 0]);
  wires:
  "IW{2,1}(1,:)'"/1 -> dotprod1/1
  "ad{2,1}"/1 -> dotprod1/2, dotprod2/2, dotprod3/2, dotprod4/2, dotprod5/2, dotprod6/2, dotprod7/2, dotprod8/2, dotprod9/2, dotprod10/2, dotprod11/2, dotprod12/2, dotprod13/2, dotprod14/2, dotprod15/2, dotprod16/2, dotprod17/2, dotprod18/2, dotprod19/2, dotprod20/2
  dotprod1/1 -> Mux/1
  "IW{2,1}(2,:)'"/1 -> dotprod2/1
  dotprod2/1 -> Mux/2
  "IW{2,1}(3,:)'"/1 -> dotprod3/1
  dotprod3/1 -> Mux/3
  "IW{2,1}(4,:)'"/1 -> dotprod4/1
  dotprod4/1 -> Mux/4
  "IW{2,1}(5,:)'"/1 -> dotprod5/1
  dotprod5/1 -> Mux/5
  "IW{2,1}(6,:)'"/1 -> dotprod6/1
  dotprod6/1 -> Mux/6
  "IW{2,1}(7,:)'"/1 -> dotprod7/1
  dotprod7/1 -> Mux/7
  "IW{2,1}(8,:)'"/1 -> dotprod8/1
  dotprod8/1 -> Mux/8
  "IW{2,1}(9,:)'"/1 -> dotprod9/1
  dotprod9/1 -> Mux/9
  "IW{2,1}(10,:)'"/1 -> dotprod10/1
  dotprod10/1 -> Mux/10
  "IW{2,1}(11,:)'"/1 -> dotprod11/1
  dotprod11/1 -> Mux/11
  "IW{2,1}(12,:)'"/1 -> dotprod12/1
  dotprod12/1 -> Mux/12
  "IW{2,1}(13,:)'"/1 -> dotprod13/1
  dotprod13/1 -> Mux/13
  "IW{2,1}(14,:)'"/1 -> dotprod14/1
  dotprod14/1 -> Mux/14
  "IW{2,1}(15,:)'"/1 -> dotprod15/1
  dotprod15/1 -> Mux/15
  "IW{2,1}(16,:)'"/1 -> dotprod16/1
  dotprod16/1 -> Mux/16
  "IW{2,1}(17,:)'"/1 -> dotprod17/1
  dotprod17/1 -> Mux/17
  "IW{2,1}(18,:)'"/1 -> dotprod18/1
  dotprod18/1 -> Mux/18
  "IW{2,1}(19,:)'"/1 -> dotprod19/1
  dotprod19/1 -> Mux/19
  "IW{2,1}(20,:)'"/1 -> dotprod20/1
  dotprod20/1 -> Mux/20
  Mux/1 -> "lz{2,1}"/1

== system ackerman_ROS_neural_controller_v2/casi 3 - 15 20 15/Layer 3/Delays 1 ==
  "p{3}" : Inport  PortDimensions=20  SampleTime=0.1
      mask Display: e = 0.06;c1 = [120 230 180]/255;c2 = ([120 230 180]+0)/(256+128);c3 = ([120 230 180]+128)/(256+128);patch([0 1 1 0],[0 0 1 1],c1);patch([0 1 1 1-e 1-e 0+e],[0 0 1 1-e 0+e 0+e],c2);patch([0 0 1 1-e 0+e 0+e],[0 1 1 1-e 1-e 0+e],c3);plot([0 1 1 0 0],[0 0 1 1 0]);
  mux : Mux  Inputs=1
      mask Display: e = 0.06;c1 = [120 150 230]/255;c2 = ([120 150 230]+0)/383;c3 = ([120 150 230]+128)/383;patch([0 1 1 0],[0 0 1 1],c1);patch([0 1 1 1-e 1-e 0+e],[0 0 1 1-e 0+e 0+e],c2);patch([0 0 1 1-e 0+e 0+e],[0 1 1 1-e 1-e 0+e],c3);plot([0 1 1 0 0],[0 0 1 1 0]);disp('Mux')
  "pd{3,2}" : Outport
      mask Display: e = 0.06;c1 = [120 230 180]/255;c2 = ([120 230 180]+0)/(256+128);c3 = ([120 230 180]+128)/(256+128);patch([0 1 1 0],[0 0 1 1],c1);patch([0 1 1 1-e 1-e 0+e],[0 0 1 1-e 0+e 0+e],c2);patch([0 0 1 1-e 0+e 0+e],[0 1 1 1-e 1-e 0+e],c3);plot([0 1 1 0 0],[0 0 1 1 0]);
  wires:
  "p{3}"/1 -> mux/1
  mux/1 -> "pd{3,2}"/1
